simulink model "bh_motor_for_param_estimation"  (R2016a)
settings: Solver=ode23s  StartTime=0.0  StopTime=10  FixedStep=0.001  RelTol=1e-5
values from neighbouring files (symbols this model uses):
  J = mot_params_TAB{'J', 'Value'}    [bh_utility_for_motor_calib.m]
  L = mot_params_TAB{'L', 'Value'}    [bh_get_motor_params.m]    (also in bh_utility_for_motor_calib.m)
  R = mot_params_TAB{'R', 'Value'}    [bh_get_motor_params.m]    (also in bh_utility_for_motor_calib.m)
  ts = T(2) - T(1)    [bh_utility_for_motor_calib.m]
undefined symbols (not defined in the file): b, Ka, Ke
settings Model: Creator=bhorton  LastModifiedBy=bhorton
settings DataIOCC: SaveOutput=off  SignalLogging=off  DSMLogging=off  VisualizeSimOutput=off  SaveTime=off
settings DebuggingCC: AlgebraicLoopMsg=error  AllowSymbolicDim=off
settings ModelReferenceCC: PropagateSignalLabelsOutOfModel=off
settings GRTTargetCC: GeneratePreprocessorConditionals=Use local settings

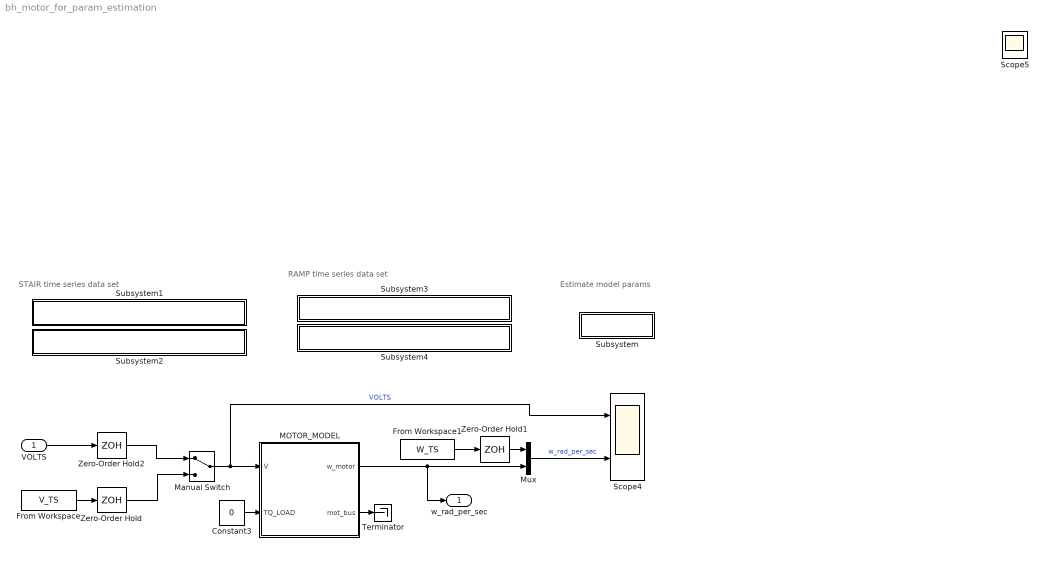
== system bh_motor_for_param_estimation ==
  note: Estimate model params
  note: STAIR time series data set
  note: RAMP time series data set
  VOLTS : Inport
  Constant3 : Constant  Value=0
  From Workspace : FromWorkspace  VariableName=V_TS  SampleTime=0  OutputAfterFinalValue=Holding final value
  From Workspace1 : FromWorkspace  VariableName=W_TS  SampleTime=0  OutputAfterFinalValue=Holding final value
  MOTOR_MODEL : Subsystem  mask(DC motor){K=Ka, B=b, J=J, GearRatio=1, R=R, L=L, Kb=Ke, ID=0}
      mask prompts: K "Torque constant (N.m/A)"; B "Viscous friction co-efficient (N.m.s)"; J "Rotor Inertia (kg.m^2)"; GearRatio "Gear ratio (w_motor/w_wheel)"; R "Armature resistance (ohms)"; L "Armature Inductance (Henry)"; Kb "Back Emf constant (V.sec/rad)"; ID "Motor_ID  (#1 to #4)"
      mask help: DC motor
      mask Display: disp('DC motor')
  Manual Switch : ManualSwitch
  Mux : Mux  Inputs=2
  Scope4 : Scope  NumInputPorts=2
  Subsystem : Subsystem
      settings: OpenFcn=spetool('bh_spesession.mat')
      mask Display: disp('ESTIMATE')
  Subsystem1 : Subsystem
      settings: OpenFcn=bh_utility_for_motor_calib( 'LOAD_INIT_AND_STAIRS' )
      mask Display: disp('Load INITIAL params with STAIRS')
  Subsystem2 : Subsystem
      settings: OpenFcn=bh_utility_for_motor_calib( 'LOAD_FINAL_AND_STAIRS' )
      mask Display: disp('Load FINAL params with STAIRS')
  Subsystem3 : Subsystem
      settings: OpenFcn=bh_utility_for_motor_calib( 'LOAD_INIT_AND_RAMPS' )
      mask Display: disp('Load INITIAL params with RAMPS')
  Subsystem4 : Subsystem
      settings: OpenFcn=bh_utility_for_motor_calib( 'LOAD_FINAL_AND_RAMPS' )
      mask Display: disp('Load FINAL params with RAMPS')
  Terminator : Terminator
  Zero-Order Hold : ZeroOrderHold  SampleTime=ts
  Zero-Order Hold1 : ZeroOrderHold  SampleTime=ts
  Zero-Order Hold2 : ZeroOrderHold  SampleTime=ts
  w_rad_per_sec : Outport
  Scope5 : Scope
  wires:
  Constant3/1 -> MOTOR_MODEL/2(TQ_LOAD)
  From Workspace/1 -> Zero-Order Hold/1
  MOTOR_MODEL/2(mot_bus) -> Terminator/1
  MOTOR_MODEL/1(w_motor) -> Mux/2, w_rad_per_sec/1
  From Workspace1/1 -> Zero-Order Hold1/1
  Mux/1 -> Scope4/2  "w_rad_per_sec"
  Zero-Order Hold1/1 -> Mux/1
  Manual Switch/1 -> Scope4/1, MOTOR_MODEL/1(V)  "VOLTS"
  Zero-Order Hold/1 -> Manual Switch/2
  VOLTS/1 -> Zero-Order Hold2/1
  Zero-Order Hold2/1 -> Manual Switch/1

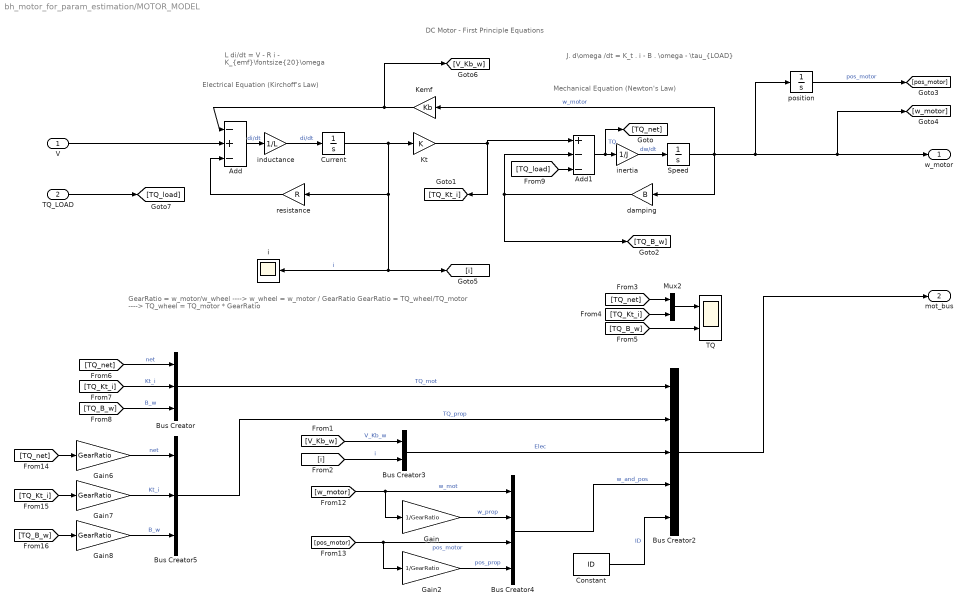
== system bh_motor_for_param_estimation/MOTOR_MODEL ==
  note: Electrical Equation
      | (Kirchoff's Law)
  note: DC Motor - First Principle Equations
  note: J. d\omega /dt = K_t . i - B . \omega - \tau_{LOAD}
  note: L di/dt = V - R i - K_{emf}\fontsize{20}\omega
  note: Mechanical Equation
      | (Newton's Law)
  note: GearRatio = w_motor/w_wheel    ---->   w_wheel = w_motor / GearRatio
      |
      | GearRatio = TQ_wheel/TQ_motor  ---->  TQ_wheel = TQ_motor * GearRatio
  V : Inport
  TQ_LOAD : Inport  Port=2
  Add : Sum  Inputs=-+-
  Add1 : Sum  Inputs=+--
  Bus Creator : BusCreator  Inputs=3
  Bus Creator2 : BusCreator  Inputs=5
  Bus Creator3 : BusCreator  Inputs=2
  Bus Creator4 : BusCreator  Inputs=4
  Bus Creator5 : BusCreator  Inputs=3
  Constant : Constant  Value=ID
  Current : Integrator
  Gain : Gain  Gain=1/GearRatio
  Gain2 : Gain  Gain=1/GearRatio
  Gain6 : Gain  Gain=GearRatio
  Gain7 : Gain  Gain=GearRatio
  Gain8 : Gain  Gain=GearRatio
  Kemf : Gain  Gain=Kb
  Kt : Gain  Gain=K
  Mux2 : Mux  Inputs=2
  Speed : Integrator
  TQ : Scope  NumInputPorts=2
  damping : Gain  Gain=B
  i : Scope
  inductance : Gain  Gain=1/L
  inertia : Gain  Gain=1/J
  position : Integrator
  resistance : Gain  Gain=R
  w_motor : Outport
  mot_bus : Outport  Port=2
  wires:
  Constant/1 -> Bus Creator2/5  "ID"
  V/1 -> Add/2
  [TQ_load] -> Add1/3
  TQ_LOAD/1 -> [TQ_load]
  [TQ_B_w] -> Gain8/1
  [TQ_Kt_i] -> Gain7/1
  Gain7/1 -> Bus Creator5/2  "Kt_i"
  Gain8/1 -> Bus Creator5/3  "B_w"
  Gain6/1 -> Bus Creator5/1  "net"
  [TQ_net] -> Gain6/1
  Bus Creator2/1 -> mot_bus/1
  Bus Creator3/1 -> Bus Creator2/3  "Elec"
  Bus Creator4/1 -> Bus Creator2/4  "w_and_pos"
  Bus Creator5/1 -> Bus Creator2/2  "TQ_prop"
  Gain2/1 -> Bus Creator4/4  "pos_prop"
  [pos_motor] -> Bus Creator4/3, Gain2/1  "pos_motor"
  Gain/1 -> Bus Creator4/2  "w_prop"
  [w_motor] -> Bus Creator4/1, Gain/1  "w_mot"
  [V_Kb_w] -> Bus Creator3/1  "V_Kb_w"
  [i] -> Bus Creator3/2  "i"
  Bus Creator/1 -> Bus Creator2/1  "TQ_mot"
  [TQ_Kt_i] -> Bus Creator/2  "Kt_i"
  [TQ_B_w] -> Bus Creator/3  "B_w"
  [TQ_net] -> Bus Creator/1  "net"
  [TQ_B_w] -> TQ/2
  [TQ_Kt_i] -> Mux2/2
  [TQ_net] -> Mux2/1
  Mux2/1 -> TQ/1
  position/1 -> [pos_motor]  "pos_motor"
  Kemf/1 -> Add/1, [V_Kb_w]
  resistance/1 -> Add/3
  Add/1 -> inductance/1  "di/dt"
  Current/1 -> i/1, [i], resistance/1, Kt/1  "i"
  Add1/1 -> inertia/1, [TQ_net]  "TQ"
  Speed/1 -> damping/1, w_motor/1, [w_motor], position/1, Kemf/1  "w_motor"
  inductance/1 -> Current/1  "di/dt"
  Kt/1 -> [TQ_Kt_i], Add1/1
  damping/1 -> Add1/2, [TQ_B_w]
  inertia/1 -> Speed/1  "dw/dt"

== system bh_motor_for_param_estimation/Subsystem ==

== system bh_motor_for_param_estimation/Subsystem1 ==

== system bh_motor_for_param_estimation/Subsystem2 ==

== system bh_motor_for_param_estimation/Subsystem3 ==

== system bh_motor_for_param_estimation/Subsystem4 ==
